simulink model "QuanserLabs_MR3003_Practice9_PartB_CDSotelo"  (R2025a)
settings: Solver=ode1  StartTime=0.0  StopTime=inf  FixedStep=0.002  RelTol=1e-3  EnableMultiTasking=on
values from neighbouring files (symbols this model uses):
  g = 9.81    [pendParam.m]
  Jp_cm = mp*Lp^2/12    (= 3.3282e-05)    [pendParam.m]
  K = place(A,B,P)    [practice9B_script.m]    (also in transformT.m = prevMatrix/T)
  kt = 0.0422    [pendParam.m]
  l = Lp/2    (= 0.0645)    [pendParam.m]
  mp = 0.024    [pendParam.m]
  mr = 0.095    [pendParam.m]
  r = 0.085    [pendParam.m]
  Rm = 7.5    [pendParam.m]
undefined symbols (not defined in the file or in its folder): HIL, qc_get_step_size
libraries: quarc_library x6, simulink x3, simulink_extras x1
settings Model: ExtModeTrigDuration=10000  Creator=A01284040  LastModifiedBy=PC-52
settings SolverCC: AlgebraicLoopSolver=TrustRegion  PositivePriorityOrder=on
settings DataIOCC: ReturnWorkspaceOutputs=off
settings DebuggingCC: UnconnectedInputMsg=warning  UnconnectedOutputMsg=warning  UnconnectedLineMsg=warning  ArithmeticOperatorsInVariantConditions=warning
settings ModelReferenceCC: EnableRefExpFcnMdlSchedulingChecks=on
settings SFSimCC: SimUseLocalCustomCode=off  CustomCodeUndefinedFunction=UseInterfaceOnly
settings RTWCC: SystemTargetFile=quarc_win64.tlc  TemplateMakefile=quarc_default_tmf  RTWUseLocalCustomCode=off  Toolchain=QUARC win64 | nmake (64-bit Windows)  BuildConfiguration=Faster Runs  GPUComputeCapability=3.5  Description=QUARC Win64 Target Using Toolchain
settings CodeAppCC: StateflowObjectComments=on
settings STFCustomTargetCC: SystemTargetFile=quarc_win64.tlc  TargetLangStandard=C99 (ISO)  MultiwordLength=2048.0  DynamicStringBufferSize=256.0  ConcurrentExecutionCompliant=on  UseToolchainInfoCompliant=on
settings GRTTargetCC: ExtMode=on  ExtModeMexFile=quarc_comm  ParMdlRefBuildCompliant=off  CompOptLevelCompliant=off  CombineOutputUpdateFcns=off  MatFileLogging=off  CPPClassGenCompliant=off  GRTInterface=on
settings ConfigComp: CovMetricSettings=dswe

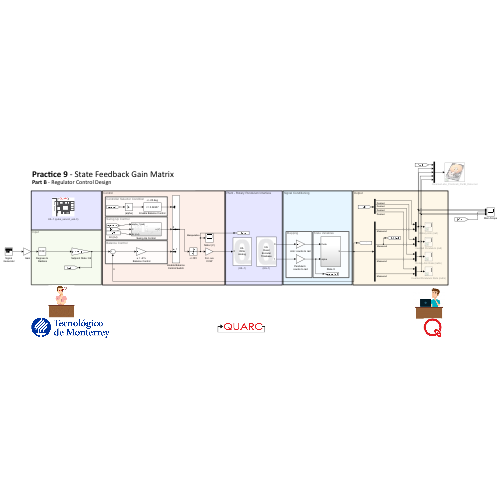
[thumbnail: Simulink's stored preview of the top-level diagram]
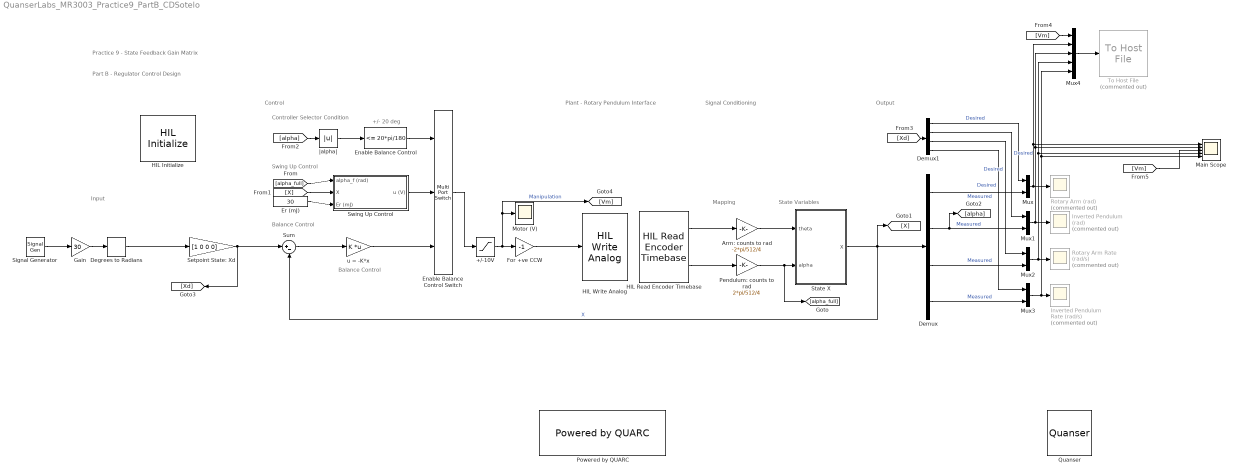
== system QuanserLabs_MR3003_Practice9_PartB_CDSotelo ==
  note: Output
  note: Mapping
  note: Controller Selector Condition
  note: Balance Control
  note: State Variables
  note: Plant - Rotary Pendulum Interface
  note: Swing Up Control
  note: Balance Control
  note: Signal Conditioning
  note: Practice 9 - State Feedback Gain Matrix
  note: Input
  note: +/- 20 deg
  note: Part B - Regulator Control Design
  note: Control
  " Gain" : Gain  Gain=30
  +/-10V : Saturate  UpperLimit=10  LowerLimit=-10
  Arm: counts to rad : Gain  Gain=-2*pi/512/4
  Degrees to Radians : simulink_extras/Transformations/Degrees to Radians
  Demux : Demux
  Demux1 : Demux
  Enable Balance Control Switch : MultiPortSwitch  DataPortOrder=Zero-based contiguous  Inputs=2  zeroidx=on  SaturateOnIntegerOverflow=off  InputSameDT=off
  Enable Balance Control : simulink/Logic and Bit Operations/Compare To Constant  relop=<=  const=20*pi/180  OutDataTypeStr=uint8  ZeroCross=off
  Er (mJ) : Constant  Value=30
  For +ve CCW : Gain  Gain=-1
  HIL Initialize : quarc_library/Data Acquisition/Generic/Configuration/HIL Initialize  object_name=HIL-1  board_type=qube_servo3_usb  board_number=0  board_options=deadband_compensation=0.65;pwm_en=0;enc0_velocity=3.0;enc1_velocity=3.0;  exclusive=off  active=on  hardware_clocks=[0]  clock_modes=[]  initial_clock_frequencies=[]  set_clock_params_at_start=off  set_clock_params_at_switch_in=off  set_clock_frequencies_at_start=off  set_clock_frequencies_at_switch_in=off  analog_input_channels=[0]  analog_input_configurations=[]  analog_input_maximums=3  analog_input_minimums=-3  set_analog_input_params_at_start=off  set_analog_input_params_at_switch_in=off  analog_output_channels=[0]  analog_output_maximums=15  analog_output_minimums=-15  initial_analog_outputs=[0]  final_analog_outputs=[0]  watchdog_analog_outputs=0  set_analog_output_params_at_start=off  set_analog_output_params_at_switch_in=off  set_analog_outputs_at_start=on  set_analog_outputs_at_switch_in=off  set_analog_outputs_at_terminate=on  set_analog_outputs_at_switch_out=off  set_analog_outputs_on_watchdog=on  digital_input_channels=[]  digital_output_channels=[0]  digital_output_configuration=[]  initial_digital_outputs=[1]  final_digital_outputs=[0]  watchdog_digital_outputs=[0]  set_digital_output_params_at_start=off  set_digital_output_params_at_switch_in=off  set_digital_outputs_at_start=on  set_digital_outputs_at_switch_in=off  set_digital_outputs_at_terminate=on  set_digital_outputs_at_switch_out=off  set_digital_outputs_on_watchdog=on  encoder_channels=[0:1]  quadrature=[4]  encoder_filter_frequency=[]  initial_encoder_counts=[0]  set_encoder_params_at_start=off  set_encoder_params_at_switch_in=off  set_encoder_counts_at_start=on  set_encoder_counts_at_switch_in=off  pwm_channels=[]  pwm_modes=[0]  pwm_frequency=23195  pwm_configuration=[1]  pwm_alignment=[0]  pwm_polarity=[1]  pwm_leading_deadband=[0]  pwm_trailing_deadband=[0]  initial_pwm_outputs=[0]  final_pwm_outputs=[0]  watchdog_pwm_outputs=[]  set_pwm_params_at_start=off  set_pwm_params_at_switch_in=off  set_pwm_outputs_at_start=off  set_pwm_outputs_at_switch_in=off  set_pwm_outputs_at_terminate=off  set_pwm_outputs_at_switch_out=off  set_pwm_outputs_on_watchdog=off  other_output_channels=[11000:11002]  initial_other_outputs=[0 1 0]  final_other_outputs=[1 0 0]  watchdog_other_outputs=[0 0 1]  set_other_outputs_at_start=on  set_other_outputs_at_switch_in=off  set_other_outputs_at_terminate=on  set_other_outputs_at_switch_out=off  set_other_outputs_on_watchdog=on
  HIL Read Encoder Timebase : quarc_library/Data Acquisition/Generic/Timebases/HIL Read Encoder Timebase  object_name=HIL-1  clock=0  channels=[0:1]  active=on  vector_output=off  data_type_mode=Inherit via back propagation  data_type=double  overflow_mode=Error on overflow  samples_in_buffer=max(ceil(1/qc_get_step_size), 1)
  HIL Write Analog : quarc_library/Data Acquisition/Generic/Immediate I//O/HIL Write Analog  object_name=HIL-1  channels=0  sample_time=-1  active=on  vector_input=off
  Inverted Pendulum (rad) : Scope  Commented=on
      settings: ActiveDisplayYMinimum=-3.92661  ActiveDisplayYMaximum=3.92354  YLabel=Inverted Pendulum Angle (rad)  DataLoggingMaxPoints=20000
  Inverted Pendulum Rate (rad/s) : Scope  Commented=on
      settings: ActiveDisplayYMinimum=-32.90866  ActiveDisplayYMaximum=29.89356  YLabel=Inverted Pendulum Angle Rate (rad/s)  DataLoggingMaxPoints=20000  DataLoggingVariableName=ScopeData2
  Main Scope : Scope  NumInputPorts=5
      settings: ActiveDisplayYMinimum=-pi  ActiveDisplayYMaximum=pi  YLabel=Rotary Arm [rad]
  Motor (V) : Scope
      settings: ActiveDisplayYMinimum=-2.91781  ActiveDisplayYMaximum=2.93828  YLabel=Motor Voltage (V)  DataLoggingMaxPoints=20000  DataLoggingVariableName=ScopeData3
  Mux{,1..3} (4 alike) : Mux  Inputs=2
  Mux4 : Mux  Inputs=5
  Pendulum: counts to rad : Gain  Gain=2*pi/512/4
  Powered by QUARC : quarc_library/Logos/Powered by QUARC
  Quanser : quarc_library/Logos/Quanser
  Rotary Arm (rad) : Scope  Commented=on
      settings: ActiveDisplayYMinimum=-1.49717  ActiveDisplayYMaximum=1.63216  YLabel=Inverted Pendulum Angle (rad)  DataLoggingMaxPoints=20000
  Rotary Arm Rate (rad/s) : Scope  Commented=on
      settings: ActiveDisplayYMinimum=-17.98454  ActiveDisplayYMaximum=14.8209  YLabel=Rotary Arm Angle Rate (rad/s)  DataLoggingMaxPoints=20000  DataLoggingVariableName=ScopeData5
  Setpoint State: Xd : Gain  Gain=[1 0 0 0]
  Signal Generator : SignalGenerator  WaveForm=square  Frequency=0.125/2
  State X : Subsystem
  Sum : Sum  Inputs=|+-
  Swing Up Control : Subsystem
  To Host File : quarc_library/Sinks/To Host/To Host File  Commented=on  source=Specify via dialog (do not evaluate)  file_name=QuanserLabs_Practice9_PartB_Data.mat  variable_name=data  decimation=1  sample_time=-1  file_format=MAT-file v.4  options=No header or footer  append=off  final_file_name=QuanserLabs_Practice9_PartB_Data.mat  encoding=Default  bitrate=2000000
  u = -K*x : Gain  Gain=K  Multiplication=Matrix(K*u)
  |alpha| : Abs  SaturateOnIntegerOverflow=off
  wires:
  Mux1/1 -> Main Scope/2, Mux4/3, Inverted Pendulum (rad)/1
  [Vm] -> Mux4/1
  Demux1/4 -> Mux3/1  "Desired"
  Mux/1 -> Rotary Arm (rad)/1, Main Scope/1, Mux4/2
  Mux2/1 -> Rotary Arm Rate (rad/s)/1, Main Scope/4, Mux4/4
  Mux4/1 -> To Host File/1
  Setpoint State: Xd/1 -> [Xd], Sum/1
  u = -K*x/1 -> Enable Balance Control Switch/3
  Enable Balance Control/1 -> Enable Balance Control Switch/1
  Demux/2 -> Mux1/2, [alpha]  "Measured"
  Sum/1 -> u = -K*x/1
  Mux3/1 -> Main Scope/5, Mux4/5, Inverted Pendulum Rate (rad/s)/1
  Demux/1 -> Mux/2  "Measured"
  Demux1/2 -> Mux1/1  "Desired"
  [alpha_full] -> Swing Up Control/1(alpha_f (rad))
  Demux1/1 -> Mux/1  "Desired"
  Demux/3 -> Mux2/2  "Measured"
  For +ve CCW/1 -> HIL Write Analog/1
  [X] -> Swing Up Control/2(X)
  Swing Up Control/1(u (V)) -> Enable Balance Control Switch/2
  [alpha] -> |alpha|/1
  Enable Balance Control Switch/1 -> +/-10V/1
  [Xd] -> Demux1/1
  Demux/4 -> Mux3/2  "Measured"
  +/-10V/1 -> [Vm], Motor (V)/1, For +ve CCW/1  "Manipulation"
  Pendulum: counts to rad/1 -> State X/2(alpha), [alpha_full]
  |alpha|/1 -> Enable Balance Control/1
  State X/1(X) -> [X], Demux/1, Sum/2  "X"
  HIL Read Encoder Timebase/1 -> Arm: counts to rad/1
  Arm: counts to rad/1 -> State X/1(theta)
  HIL Read Encoder Timebase/2 -> Pendulum: counts to rad/1
  Demux1/3 -> Mux2/1  "Desired"
  " Gain"/1 -> Degrees to Radians/1
  Er (mJ)/1 -> Swing Up Control/3(Er (mJ))
  Signal Generator/1 -> " Gain"/1
  Degrees to Radians/1 -> Setpoint State: Xd/1
  [Vm] -> Main Scope/3

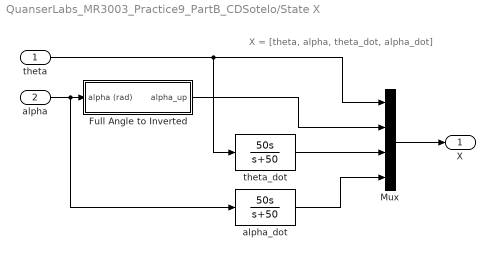
== system QuanserLabs_MR3003_Practice9_PartB_CDSotelo/State X ==
  note: X = [theta, alpha, theta_dot, alpha_dot]
  theta : Inport
  alpha : Inport  Port=2
  Full Angle to Inverted : Subsystem
  Mux : Mux
  alpha_dot : TransferFcn  Numerator=[50 0]  Denominator=[1 50]
  theta_dot : TransferFcn  Numerator=[50 0]  Denominator=[1 50]
  X : Outport  VectorParamsAs1DForOutWhenUnconnected=off
  wires:
  Mux/1 -> X/1
  alpha/1 -> alpha_dot/1, Full Angle to Inverted/1(alpha (rad))
  Full Angle to Inverted/1(alpha_up) -> Mux/2
  theta/1 -> theta_dot/1, Mux/1
  theta_dot/1 -> Mux/3
  alpha_dot/1 -> Mux/4

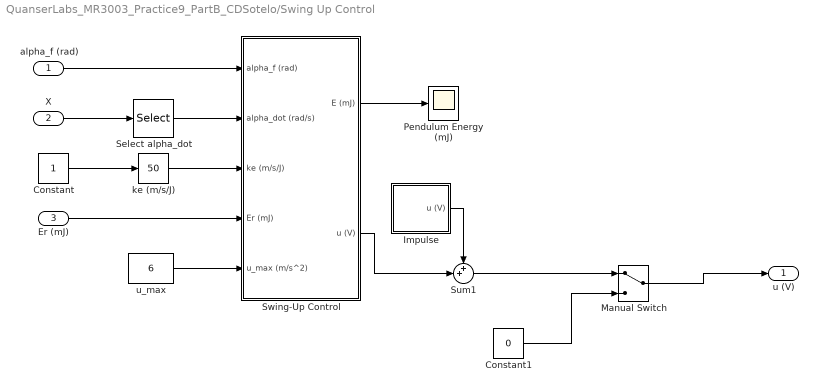
== system QuanserLabs_MR3003_Practice9_PartB_CDSotelo/Swing Up Control ==
  alpha_f (rad) : Inport
  X : Inport  Port=2
  Er (mJ) : Inport  Port=3
  Constant : Constant
  Constant1 : Constant  Value=0
  Impulse : Subsystem
  Manual Switch : ManualSwitch
  Pendulum Energy (mJ) : Scope
      settings: ActiveDisplayYMinimum=-3.96378  ActiveDisplayYMaximum=35.674  DataLoggingVariableName=ScopeData3
  Select alpha_dot : Selector  InputPortWidth=4  IndexOptions=Index vector (dialog)  Indices=[4]  OutputSizes=1
  Sum1 : Sum  Inputs=++|
  Swing-Up Control : Subsystem
  ke (m/s/J) : simulink/Math Operations/Slider Gain  gain=50  low=0  high=100
  u_max : Constant  Value=6
  u (V) : Outport
  wires:
  u_max/1 -> Swing-Up Control/5(u_max (m/s^2))
  Er (mJ)/1 -> Swing-Up Control/4(Er (mJ))
  Swing-Up Control/1(E (mJ)) -> Pendulum Energy (mJ)/1
  X/1 -> Select alpha_dot/1
  Constant/1 -> ke (m/s/J)/1
  Select alpha_dot/1 -> Swing-Up Control/2(alpha_dot (rad/s))
  Swing-Up Control/2(u (V)) -> Sum1/2
  Impulse/1(u (V)) -> Sum1/1
  ke (m/s/J)/1 -> Swing-Up Control/3(ke (m/s/J))
  alpha_f (rad)/1 -> Swing-Up Control/1(alpha_f (rad))
  Manual Switch/1 -> u (V)/1
  Sum1/1 -> Manual Switch/1
  Constant1/1 -> Manual Switch/2

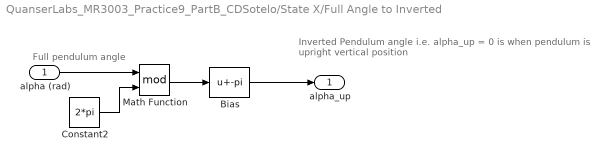
== system QuanserLabs_MR3003_Practice9_PartB_CDSotelo/State X/Full Angle to Inverted ==
  note: Inverted Pendulum angle
      | i.e. alpha_up = 0 is when pendulum is upright vertical position
  note: Full pendulum angle
  alpha (rad) : Inport
  Bias : Bias  Bias=-pi  SaturateOnIntegerOverflow=off
  Constant2 : Constant  Value=2*pi
  Math Function : Math  Operator=mod  SignedPower=on
  alpha_up : Outport  VectorParamsAs1DForOutWhenUnconnected=off
  wires:
  Constant2/1 -> Math Function/2
  alpha (rad)/1 -> Math Function/1
  Bias/1 -> alpha_up/1
  Math Function/1 -> Bias/1

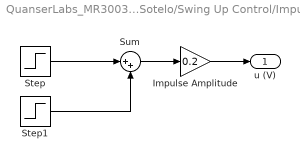
== system QuanserLabs_MR3003_Practice9_PartB_CDSotelo/Swing Up Control/Impulse ==
  Impulse Amplitude : Gain  Gain=0.2
  Step : Step  SampleTime=0
  Step1 : Step  Time=1.1  After=-1  SampleTime=0
  Sum : Sum  Inputs=|++
  u (V) : Outport  VectorParamsAs1DForOutWhenUnconnected=off
  wires:
  Step1/1 -> Sum/2
  Step/1 -> Sum/1
  Sum/1 -> Impulse Amplitude/1
  Impulse Amplitude/1 -> u (V)/1

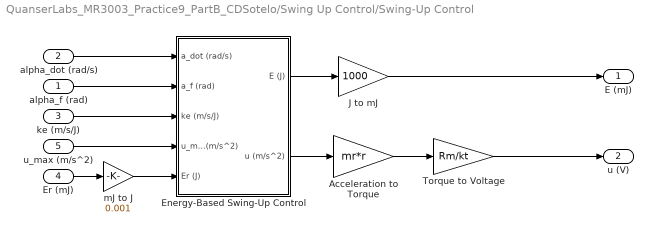
== system QuanserLabs_MR3003_Practice9_PartB_CDSotelo/Swing Up Control/Swing-Up Control ==
  alpha_f (rad) : Inport
  alpha_dot (rad/s) : Inport  Port=2
  ke (m/s/J) : Inport  Port=3
  Er (mJ) : Inport  Port=4
  u_max (m/s^2) : Inport  Port=5
  Acceleration to Torque : Gain  Gain=mr*r
  Energy-Based Swing-Up Control : Subsystem
  J to mJ : Gain  Gain=1000
  Torque to Voltage : Gain  Gain=Rm/kt
  mJ to J : Gain  Gain=0.001
  E (mJ) : Outport  VectorParamsAs1DForOutWhenUnconnected=off
  u (V) : Outport  Port=2  VectorParamsAs1DForOutWhenUnconnected=off
  wires:
  Energy-Based Swing-Up Control/2(u (m/s^2)) -> Acceleration to Torque/1
  Energy-Based Swing-Up Control/1(E (J)) -> J to mJ/1
  alpha_f (rad)/1 -> Energy-Based Swing-Up Control/2(a_f (rad))
  ke (m/s/J)/1 -> Energy-Based Swing-Up Control/3(ke (m/s/J))
  u_max (m/s^2)/1 -> Energy-Based Swing-Up Control/4(u_max (m/s^2))
  Acceleration to Torque/1 -> Torque to Voltage/1
  Er (mJ)/1 -> mJ to J/1
  J to mJ/1 -> E (mJ)/1
  Torque to Voltage/1 -> u (V)/1
  alpha_dot (rad/s)/1 -> Energy-Based Swing-Up Control/1(a_dot (rad/s))
  mJ to J/1 -> Energy-Based Swing-Up Control/5(Er (J))

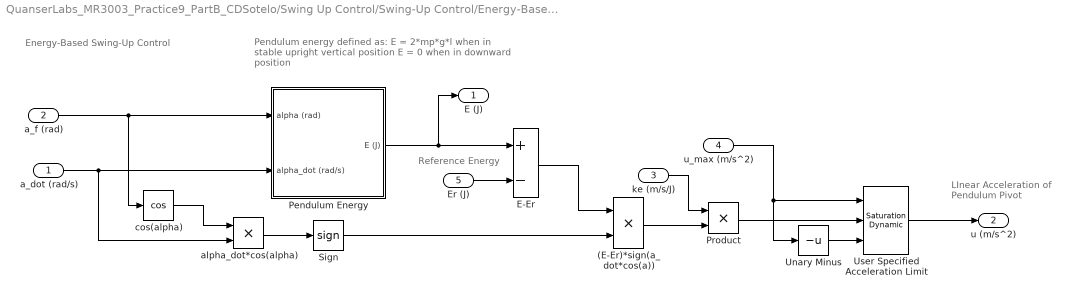
== system QuanserLabs_MR3003_Practice9_PartB_CDSotelo/Swing Up Control/Swing-Up Control/Energy-Based Swing-Up Control ==
  note: Energy-Based Swing-Up Control
  note: LInear Acceleration of
      | Pendulum Pivot
  note: Reference Energy
  note: Pendulum energy defined as:
      | E = 2*mp*g*l when in stable upright vertical position
      | E = 0 when in downward position
  a_dot (rad/s) : Inport
  a_f (rad) : Inport  Port=2
  ke (m/s/J) : Inport  Port=3
  u_max (m/s^2) : Inport  Port=4
  Er (J) : Inport  Port=5
  (E-Er)*sign(a_dot*cos(a)) : Product  RndMeth=Zero
  E-Er : Sum  Inputs=+-
  Pendulum Energy : Subsystem
  Product : Product  RndMeth=Zero
  Sign : Signum
  Unary Minus : UnaryMinus
  User Specified Acceleration Limit : simulink/Discontinuities/Saturation Dynamic  OutMin=[]  OutMax=[]  OutDataTypeStr=Inherit: Same as second input  OutDataType=fixdt(1, 16)  OutScaling=2^-10  DoSatur=off
  alpha_dot*cos(alpha) : Product  RndMeth=Zero
  cos(alpha) : Trigonometry  Operator=cos
  E (J) : Outport  VectorParamsAs1DForOutWhenUnconnected=off
  u (m/s^2) : Outport  Port=2  VectorParamsAs1DForOutWhenUnconnected=off
  wires:
  a_f (rad)/1 -> Pendulum Energy/1(alpha (rad)), cos(alpha)/1
  Sign/1 -> (E-Er)*sign(a_dot*cos(a))/2
  alpha_dot*cos(alpha)/1 -> Sign/1
  cos(alpha)/1 -> alpha_dot*cos(alpha)/1
  E-Er/1 -> (E-Er)*sign(a_dot*cos(a))/1
  Pendulum Energy/1(E (J)) -> E (J)/1, E-Er/1
  a_dot (rad/s)/1 -> alpha_dot*cos(alpha)/2, Pendulum Energy/2(alpha_dot (rad/s))
  (E-Er)*sign(a_dot*cos(a))/1 -> Product/2
  Er (J)/1 -> E-Er/2
  ke (m/s/J)/1 -> Product/1
  Product/1 -> User Specified Acceleration Limit/2
  u_max (m/s^2)/1 -> User Specified Acceleration Limit/1, Unary Minus/1
  Unary Minus/1 -> User Specified Acceleration Limit/3
  User Specified Acceleration Limit/1 -> u (m/s^2)/1

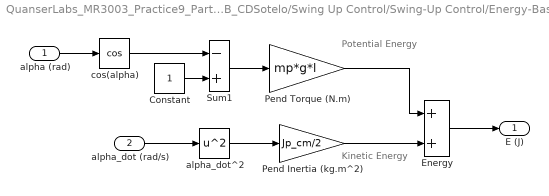
== system QuanserLabs_MR3003_Practice9_PartB_CDSotelo/Swing Up Control/Swing-Up Control/Energy-Based Swing-Up Control/Pendulum Energy ==
  note: Kinetic Energy
  note: Potential Energy
  alpha (rad) : Inport
  alpha_dot (rad/s) : Inport  Port=2
  Constant : Constant
  Energy : Sum  SaturateOnIntegerOverflow=on
  Pend Inertia (kg.m^2) : Gain  Gain=Jp_cm/2
  Pend Torque (N.m) : Gain  Gain=mp*g*l
  Sum1 : Sum  Inputs=-+  SaturateOnIntegerOverflow=on
  alpha_dot^2 : Math  Operator=square  SignedPower=on
  cos(alpha) : Trigonometry  Operator=cos
  E (J) : Outport  VectorParamsAs1DForOutWhenUnconnected=off
  wires:
  Sum1/1 -> Pend Torque (N.m)/1
  Constant/1 -> Sum1/2
  Pend Inertia (kg.m^2)/1 -> Energy/2
  alpha_dot^2/1 -> Pend Inertia (kg.m^2)/1
  Pend Torque (N.m)/1 -> Energy/1
  alpha (rad)/1 -> cos(alpha)/1
  alpha_dot (rad/s)/1 -> alpha_dot^2/1
  Energy/1 -> E (J)/1
  cos(alpha)/1 -> Sum1/1
